simulink model "TestFMU"  (R2020b)
settings: Solver=FixedStepAuto  StartTime=0.0  StopTime=10.0  FixedStep=0.001  RelTol=1e-3
undefined symbols (not defined in the file or in its folder): DCHigh, DCLow
libraries: fl_lib x2, nesl_utility x2
settings Model: DataDictionary=FMUBus.sldd  Creator=cao2851  LastModifiedBy=cao2851

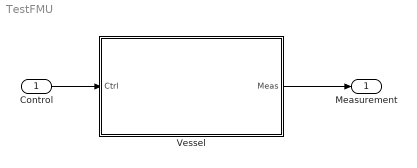
== system TestFMU ==
  Control : Inport  OutDataTypeStr=Bus: Control
  Vessel : Subsystem
  Measurement : Outport  OutDataTypeStr=Bus: Measurement
  wires:
  Control/1 -> Vessel/1(Ctrl)
  Vessel/1(Meas) -> Measurement/1

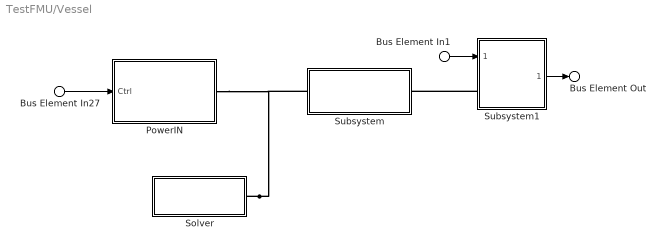
== system TestFMU/Vessel ==
  Bus Element In27 : Inport  PortName=Ctrl  Element=InputVoltage
  Bus Element In1 : Inport  PortName=Ctrl  Element=PowerLoad
  PowerIN : Subsystem
  Solver : Subsystem
  Subsystem : Subsystem  ReferencedSubsystem=Line
  Subsystem1 : Subsystem  ReferencedSubsystem=Load
  Bus Element Out : Outport  PortName=Meas  Element=PowerLoad
  wires:
  Subsystem1/1 -> Bus Element Out/1
  Bus Element In27/1 -> PowerIN/1(Ctrl)
  Bus Element In1/1 -> Subsystem1/1
  connections:
  Solver/RConn1 -- PowerIN/RConn1 -- Subsystem/LConn1
  Subsystem1/LConn1 -- Subsystem/RConn1

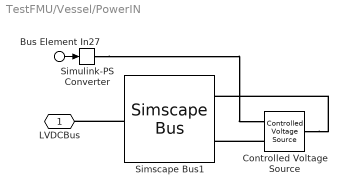
== system TestFMU/Vessel/PowerIN ==
  Bus Element In27 : Inport  PortName=Ctrl  Element=LoadSetpoint
  Controlled Voltage Source : fl_lib/Electrical/Electrical Sources/Controlled Voltage Source
  Simscape Bus1 : SimscapeBus  HierarchyStrings=DCHigh;DCLow
  Simulink-PS Converter : nesl_utility/Simulink-PS Converter  PhysicalDomain=network_engine_domain  SubClassName=ps_input  LeftPortType=input  RightPortType=output  PseudoPeriodic=off  Frequencies=[]  NoiseDistribution=none  NoiseParameters=[]  Unit=1  AffineConversion=off  FilteringAndDerivatives=provide  SimscapeFilterOrder=1  InputFilterTimeConstant=0.001  UdotUserProvided=0
  LVDCBus : PMIOPort  Side=Right
  wires:
  Bus Element In27/1 -> Simulink-PS Converter/1
  connections:
  Simscape Bus1/RConn1 -- LVDCBus/RConn1
  Simulink-PS Converter/RConn1 -- Controlled Voltage Source/RConn1
  Controlled Voltage Source/LConn1 -- Simscape Bus1/LConn1
  Controlled Voltage Source/RConn2 -- Simscape Bus1/LConn2

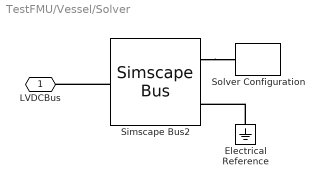
== system TestFMU/Vessel/Solver ==
  Electrical Reference : fl_lib/Electrical/Electrical Elements/Electrical Reference
  Simscape Bus2 : SimscapeBus  HierarchyStrings=DCHigh;DCLow
  Solver Configuration : nesl_utility/Solver Configuration  PhysicalDomain=network_engine_domain  SubClassName=solver  LeftPortType=input  RightPortType=generic  Tones=[]  Harmonics=[]  SimulateNoise=off  Profile=off  UseLocalSampling=off  EnableSwitchedLinearOptims=on  FrequencyDomain=off  UseCCode=off  RelTol=0.001  AbsTol=1e-06  MinStep=1e-09  ToWorkspace=off  RevertToSquareIcSolve=off  NumHomotopyIterations=100  PhasorMode=off  PhasorModeNumHarmonics=1  DoDC=off  ResidualTolerance=1e-09  UseLocalSolver=on  LocalSolverChoice=NE_BACKWARD_EULER_ADVANCER  LocalSolverSampleTime=Ts  DoFixedCost=on  MaxNonlinIter=3  MaxModeIter=2  ComputeImpulses=off  ImpulseIterations=2  LinearAlgebra=auto  EquationFormulation=NE_TIME_EF  DelaysMemoryBudget=1024  AutomaticFiltering=off  FilteringTimeConstant=0.001  PartitionStorageMethod=AS_NEEDED  PartitionMemoryBudget=1024  PartitionMethod=ROBUST
      settings: SourceProductBaseCode=PW,SS
  LVDCBus : PMIOPort  Side=Right
  connections:
  Simscape Bus2/RConn1 -- LVDCBus/RConn1
  Simscape Bus2/LConn1 -- Solver Configuration/RConn1
  Electrical Reference/LConn1 -- Simscape Bus2/LConn2
